simulink model "FSM"  (R2024b)
settings: Solver=FixedStepDiscrete  StartTime=0.0  StopTime=10.0  FixedStep=0.1  RelTol=1e-3  EnableMultiTasking=on
settings Model: Creator=jacob  LastModifiedBy=jacob
settings SolverCC: AlgebraicLoopSolver=TrustRegion  AutoInsertRateTranBlk=on
settings DataIOCC: LimitDataPoints=on
settings OptimizationCC: LifeSpan=inf
settings DebuggingCC: UnconnectedInputMsg=warning  UnconnectedOutputMsg=warning  UnconnectedLineMsg=warning  AllowSymbolicDim=off  SFUnexpectedBacktrackingDiag=warning  SFNoUnconditionalDefaultTransitionDiag=warning  SFExecutionAtInitializationDiag=none  ArithmeticOperatorsInVariantConditions=warning
settings ModelReferenceCC: EnableRefExpFcnMdlSchedulingChecks=on
settings SFSimCC: SimUseLocalCustomCode=off  CustomCodeUndefinedFunction=UseInterfaceOnly
settings RTWCC: RTWUseLocalCustomCode=off  GPUComputeCapability=3.5  DLArmComputeVersion=19.05
settings CodeAppCC: StateflowObjectComments=on
settings GRTTargetCC: TargetLangStandard=C89/C90 (ANSI)
settings ConfigComp: CovMetricSettings=dw  CovSaveCumulativeToWorkspaceVar=on  CovSaveSingleToWorkspaceVar=on  CovExternalEMLEnable=off

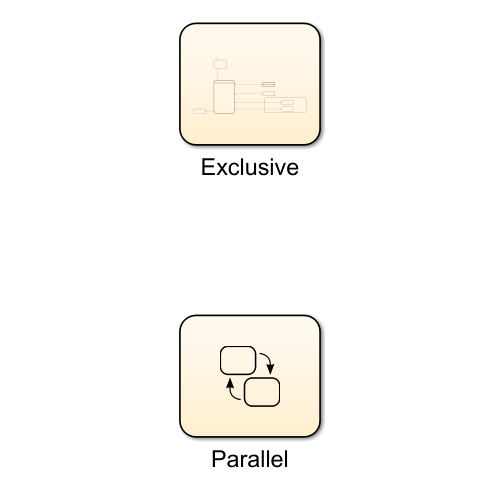
[thumbnail: Simulink's stored preview of the top-level diagram]
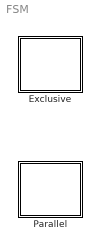
== system FSM ==
  Exclusive : Stateflow chart  TreatAsAtomicUnit=on
  Parallel : Stateflow chart  TreatAsAtomicUnit=on

== stateflow chart FSM/Exclusive ==
  state Initialization
  state ObjectDetection
    state DetectObject
    state Rotate
    state IdentifyColor
    state EstimateObjLocation
    state NoObject
    state IdentifyGender
    state LocateCustomer
    DetectObject -> Rotate [order 1] : [class=='none']
    Rotate -> DetectObject
    (default) -> (junction 19)
    DetectObject -> 135 [order 4] : [timeout]
    (junction 136) -> 135
    IdentifyColor -> IdentifyColor [order 1] : [color == 'red']
    (junction 19) -> DetectObject [order 1] : [obj]
    (junction 19) -> NoObject [order 2]
    DetectObject -> IdentifyColor [order 6] : [class=='traffic_light']
    IdentifyColor -> (junction 136) [order 2] : [color=='green']{goal='ingredients'}
    (junction 94) -> (junction 136)
    EstimateObjLocation -> (junction 94) [order 1] : [~inReach]
    DetectObject -> EstimateObjLocation [order 7] : [class=='bun']
    (junction 45) -> (junction 94)
    EstimateObjLocation -> 86 [order 2] : [inReach]
    DetectObject -> EstimateObjLocation [order 2] : [class=='patty']
    DetectObject -> IdentifyGender [order 5] : [class=='face']
    IdentifyGender -> (junction 69) : [genderIdentified]
    (junction 69) -> (junction 45) [order 1] : [image=='face']{goal='customer'}
    NoObject -> 120
    (junction 69) -> (junction 72) [order 2]
    (junction 74) -> (junction 45)
    LocateCustomer -> (junction 74) [order 1] : [~inReach]
    DetectObject -> 55 [order 3] : [class=='stop_sign']
    (junction 72) -> LocateCustomer : [image=='customer']
    LocateCustomer -> 116 [order 2] : [inReach]
  state Navigation
    state PathPlanning
    state TrajectoryPlanning
    state TrajectoryExecution
    (default) -> PathPlanning
    PathPlanning -> TrajectoryPlanning
    TrajectoryPlanning -> TrajectoryExecution
  state Idle
  state ActuateGrasper
    state Pickup
    state Deposit
  state Error
  (default) -> Initialization
  Initialization -> ObjectDetection : {obj='traffic_light'}
  28 -> Navigation
  56 -> Idle
  87 -> Pickup
  117 -> Deposit
  121 -> Error

== stateflow chart FSM/Parallel ==
  state CameraDetection [parallel]
    settings: executionOrder=1
    state IdentifyTrafficLight
    state Idle
    state IdentifyBurger
    state IdentifyGender
    (default) -> (junction 22)
    CameraDetection.Idle -> (junction 22)
    (junction 22) -> IdentifyTrafficLight [order 1] : [obj == 'TrafficLight']
    IdentifyTrafficLight -> CameraDetection.Idle
    (junction 22) -> (junction 37) [order 2]
    (junction 37) -> IdentifyBurger [order 1] : [obj == 'Burger']
    (junction 37) -> (junction 34) [order 2]
    (junction 34) -> (junction 43) : [obj == 'Face']
    (junction 43) -> IdentifyGender : [task == 'identify']
  state Navigation [parallel]
    settings: executionOrder=2
    state Idle
    state ?
    state Path & Trajectory Planning
    state Command Motors
    (default) -> Navigation.Idle
    Navigation.Idle -> ? : [lightColor == 'green']
    Path & Trajectory Planning -> Command Motors
  data: color local; init local; task local
